simulink model "controller_full"  (R2020b)
settings: Solver=VariableStepAuto  StartTime=0.0  StopTime=10.0  RelTol=1e-3
undefined symbols (not defined in the file): K_d, K_p, params, r_des
settings Model: Creator=Danil  LastModifiedBy=Danil

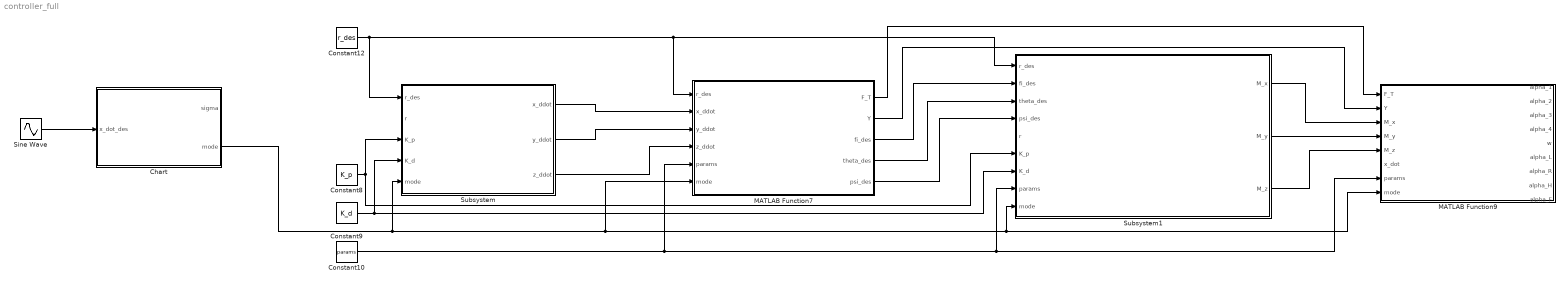
== system controller_full ==
  Chart : Stateflow chart  TreatAsAtomicUnit=on
      settings: PortSchema="{\"entries\":[{\"content\":{\"sides\":[{\"content\":{\"connectorIds\":[\"In1\"]},\"type\":\"ConnectorPlacement.EquallySpacedRectSide\",\"uuid\":\"990aaa4d-e872-427e-8bc8-a44f7de52f17\"},{\"content\":{\"connectorIds\":[\"Out2\",\"Out1\"],\"side\":\"RIGHT\"},\"type\":\"ConnectorPlacement.EquallySpacedRectSide\",\"uuid\":\"6e7ad4a8-1d47-4f26-af3c-4dfef899b5bc\"},{\"content\":{\"connectorIds\":[],\"side\":\"TOP\"},\"type\":\"ConnectorPlacement.EquallySpacedRectSide\",\"uuid\":\"20d3b10c-4783-40ca-8243-63709ccaf162\"},{\"content\":{\"connectorIds\":[],\"side\":\"HIDDEN\"},\"type\":\"ConnectorPlacement.EquallySpacedRectSide\",\"uuid\":\"c78cf433-ac9b-47b8-aa1e-24a5718d794b\"}]},\"type\":\"ConnectorPlacement.EquallySpacedConnector\",\"uuid\":\"eb598262-5703-4057-871f-faa738de211a\"}],\"packageUris\":[\"http://schema.mathworks.com/mf0/Connector/R2020b\"],\"version\":\"1.0\"}"
  Constant10 : Constant  Value=params  OutDataTypeStr=Bus: params_bus
  Constant12 : Constant  Value=r_des  OutDataTypeStr=Bus: r_des_bus
  Constant8 : Constant  Value=K_p  OutDataTypeStr=Bus: K_p_bus
  Constant9 : Constant  Value=K_d  OutDataTypeStr=Bus: K_d_bus
  MATLAB Function7 : MATLAB Function  TreatAsAtomicUnit=on
  MATLAB Function9 : MATLAB Function  TreatAsAtomicUnit=on
  Sine Wave : Sin  Amplitude=40  SampleTime=0
  Subsystem : Subsystem
  Subsystem1 : Subsystem
  wires:
  Sine Wave/1 -> Chart/1(x_dot_des)
  Subsystem1/1(M_x) -> MATLAB Function9/3(M_x)
  Subsystem1/2(M_y) -> MATLAB Function9/4(M_y)
  Subsystem1/3(M_z) -> MATLAB Function9/5(M_z)
  Constant10/1 -> MATLAB Function7/5(params), Subsystem1/8(params), MATLAB Function9/7(params)
  Constant12/1 -> Subsystem/1(r_des), MATLAB Function7/1(r_des), Subsystem1/1(r_des)
  Constant8/1 -> Subsystem/3(K_p), Subsystem1/6(K_p)
  Constant9/1 -> Subsystem/4(K_d), Subsystem1/7(K_d)
  Chart/1(mode) -> Subsystem/5(mode), MATLAB Function9/8(mode), Subsystem1/9(mode), MATLAB Function7/6(mode)
  Subsystem/1(x_ddot) -> MATLAB Function7/2(x_ddot)
  Subsystem/2(y_ddot) -> MATLAB Function7/3(y_ddot)
  Subsystem/3(z_ddot) -> MATLAB Function7/4(z_ddot)
  MATLAB Function7/5(psi_des) -> Subsystem1/4(psi_des)
  MATLAB Function7/4(theta_des) -> Subsystem1/3(theta_des)
  MATLAB Function7/3(fi_des) -> Subsystem1/2(fi_des)
  MATLAB Function7/2(Y) -> MATLAB Function9/2(Y)
  MATLAB Function7/1(F_T) -> MATLAB Function9/1(F_T)

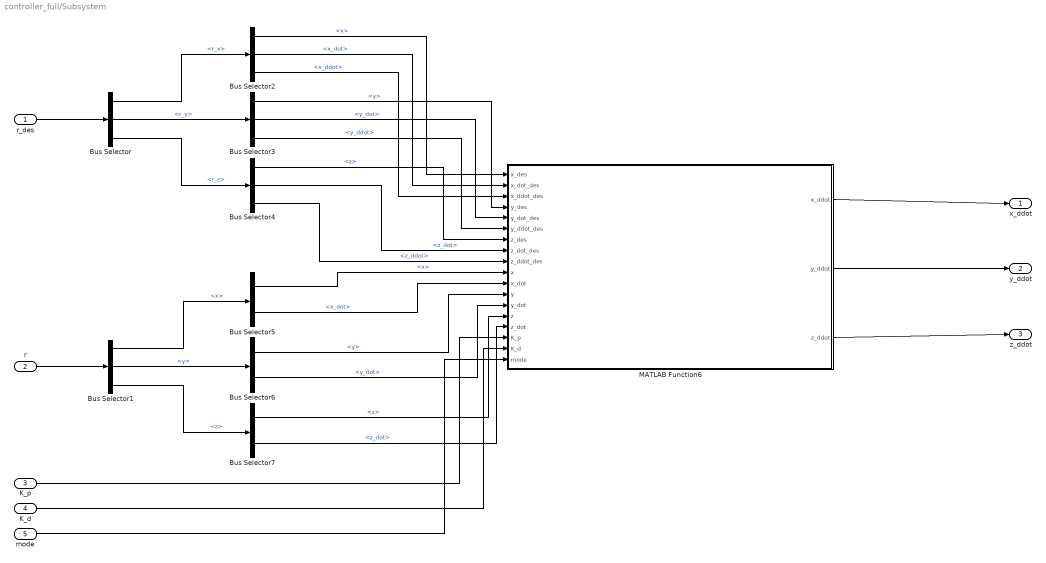
== system controller_full/Subsystem ==
  r_des : Inport
  r : Inport  Port=2
  K_p : Inport  Port=3
  K_d : Inport  Port=4
  mode : Inport  Port=5
  Bus Selector : BusSelector  OutputSignals=r_x,r_y,r_z
  Bus Selector1 : BusSelector  OutputSignals=x,y,z
  Bus Selector2 : BusSelector  OutputSignals=x,x_dot,x_ddot
  Bus Selector3 : BusSelector  OutputSignals=y,y_dot,y_ddot
  Bus Selector4 : BusSelector  OutputSignals=z,z_dot,z_ddot
  Bus Selector5 : BusSelector  OutputSignals=x,x_dot
  Bus Selector6 : BusSelector  OutputSignals=y,y_dot
  Bus Selector7 : BusSelector  OutputSignals=z,z_dot
  MATLAB Function6 : MATLAB Function  TreatAsAtomicUnit=on
  x_ddot : Outport
  y_ddot : Outport  Port=2
  z_ddot : Outport  Port=3
  wires:
  Bus Selector3/1 -> MATLAB Function6/4(y_des)  "<y>"
  Bus Selector4/3 -> MATLAB Function6/9(z_ddot_des)  "<z_ddot>"
  Bus Selector4/1 -> MATLAB Function6/7(z_des)  "<z>"
  Bus Selector/1 -> Bus Selector2/1  "<r_x>"
  Bus Selector5/2 -> MATLAB Function6/11(x_dot)  "<x_dot>"
  Bus Selector3/2 -> MATLAB Function6/5(y_dot_des)  "<y_dot>"
  Bus Selector/3 -> Bus Selector4/1  "<r_z>"
  r/1 -> Bus Selector1/1
  r_des/1 -> Bus Selector/1
  Bus Selector2/1 -> MATLAB Function6/1(x_des)  "<x>"
  Bus Selector5/1 -> MATLAB Function6/10(x)  "<x>"
  MATLAB Function6/2(y_ddot) -> y_ddot/1
  MATLAB Function6/3(z_ddot) -> z_ddot/1
  K_d/1 -> MATLAB Function6/17(K_d)
  K_p/1 -> MATLAB Function6/16(K_p)
  Bus Selector1/3 -> Bus Selector7/1  "<z>"
  Bus Selector2/2 -> MATLAB Function6/2(x_dot_des)  "<x_dot>"
  Bus Selector7/2 -> MATLAB Function6/15(z_dot)  "<z_dot>"
  MATLAB Function6/1(x_ddot) -> x_ddot/1
  Bus Selector6/1 -> MATLAB Function6/12(y)  "<y>"
  Bus Selector7/1 -> MATLAB Function6/14(z)  "<z>"
  Bus Selector4/2 -> MATLAB Function6/8(z_dot_des)  "<z_dot>"
  Bus Selector2/3 -> MATLAB Function6/3(x_ddot_des)  "<x_ddot>"
  Bus Selector1/1 -> Bus Selector5/1  "<x>"
  Bus Selector1/2 -> Bus Selector6/1  "<y>"
  Bus Selector6/2 -> MATLAB Function6/13(y_dot)  "<y_dot>"
  Bus Selector3/3 -> MATLAB Function6/6(y_ddot_des)  "<y_ddot>"
  Bus Selector/2 -> Bus Selector3/1  "<r_y>"
  mode/1 -> MATLAB Function6/18(mode)

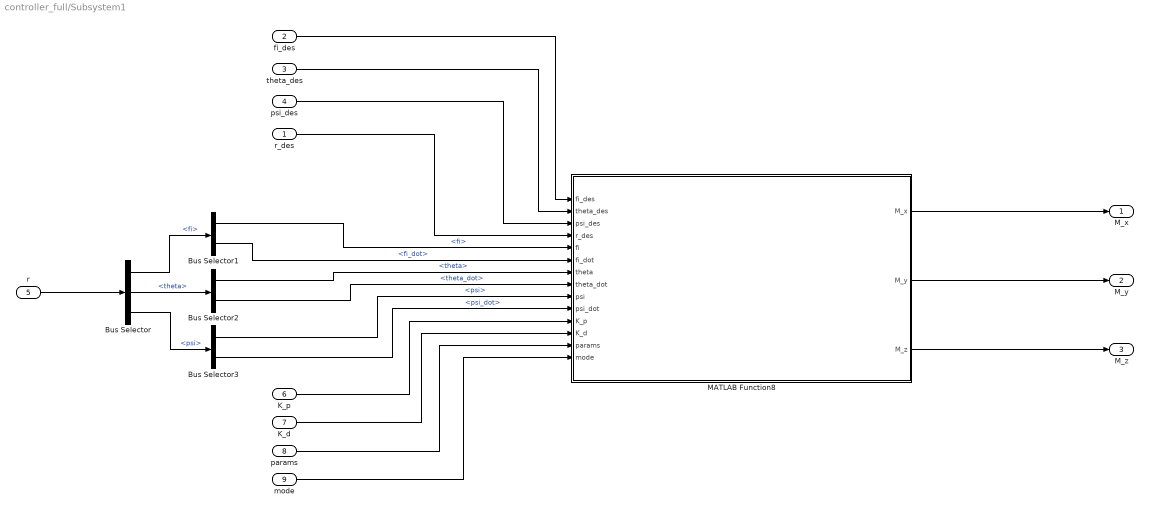
== system controller_full/Subsystem1 ==
  r_des : Inport
  fi_des : Inport  Port=2
  theta_des : Inport  Port=3
  psi_des : Inport  Port=4
  r : Inport  Port=5
  K_p : Inport  Port=6
  K_d : Inport  Port=7
  params : Inport  Port=8
  mode : Inport  Port=9
  Bus Selector : BusSelector  OutputSignals=fi,theta,psi
  Bus Selector1 : BusSelector  OutputSignals=fi,fi_dot
  Bus Selector2 : BusSelector  OutputSignals=theta,theta_dot
  Bus Selector3 : BusSelector  OutputSignals=psi,psi_dot
  MATLAB Function8 : MATLAB Function  TreatAsAtomicUnit=on
  M_x : Outport
  M_y : Outport  Port=2
  M_z : Outport  Port=3
  wires:
  Bus Selector3/1 -> MATLAB Function8/9(psi)  "<psi>"
  Bus Selector1/2 -> MATLAB Function8/6(fi_dot)  "<fi_dot>"
  Bus Selector/1 -> Bus Selector1/1  "<fi>"
  Bus Selector1/1 -> MATLAB Function8/5(fi)  "<fi>"
  r/1 -> Bus Selector/1
  MATLAB Function8/3(M_z) -> M_z/1
  MATLAB Function8/1(M_x) -> M_x/1
  MATLAB Function8/2(M_y) -> M_y/1
  Bus Selector2/2 -> MATLAB Function8/8(theta_dot)  "<theta_dot>"
  K_p/1 -> MATLAB Function8/11(K_p)
  Bus Selector2/1 -> MATLAB Function8/7(theta)  "<theta>"
  Bus Selector/2 -> Bus Selector2/1  "<theta>"
  r_des/1 -> MATLAB Function8/4(r_des)
  params/1 -> MATLAB Function8/13(params)
  psi_des/1 -> MATLAB Function8/3(psi_des)
  fi_des/1 -> MATLAB Function8/1(fi_des)
  K_d/1 -> MATLAB Function8/12(K_d)
  theta_des/1 -> MATLAB Function8/2(theta_des)
  Bus Selector3/2 -> MATLAB Function8/10(psi_dot)  "<psi_dot>"
  Bus Selector/3 -> Bus Selector3/1  "<psi>"
  mode/1 -> MATLAB Function8/14(mode)

== matlab function controller_full/MATLAB Function9 ==
  data: alpha_1 output; alpha_2 output; alpha_3 output; alpha_4 output; F_T input; Y input; w output; M_x input; M_y input; M_z input; x_dot input; params input; alpha_L output; alpha_R output; alpha_H output; alpha_F output; mode input
function [alpha_1, alpha_2, alpha_3, alpha_4, w, alpha_L, alpha_R, alpha_H, alpha_F] = fcn(F_T, Y, M_x, M_y, M_z, x_dot, params, mode)

if mode == 0
    
    alpha_1 = (1 / (4 * params.k_Y)) * (F_T + M_x + M_y + M_z) - 7;
    alpha_2 = (1 / (4 * params.k_Y)) * (F_T + M_x - M_y - M_z);
    alpha_3 = (1 / (4 * params.k_Y)) * (F_T - M_x + M_y - M_z) - 7;
    alpha_4 = (1 / (4 * params.k_Y)) * (F_T - M_x - M_y + M_z);
    
    w = params.w_0;
    alpha_L = -7;
    alpha_R = -7;
    alpha_H = 0;
    alpha_F = 0;
    
elseif mode == 1
    
    alpha_1 = 7.5;
    alpha_2 = 7.5;
    alpha_3 = 7.5;
    alpha_4 = 7.5;

    w = (50000 * F_T + 245100) / 77;

    alpha_L = (500 * M_x + 500 * Y + 102201 * params.S_k * params.rho - 14630 * params.S_k * params.rho * x_dot) / (30 * params.S_k * params.rho * (70 * x_dot - 489));
    alpha_R = - (500 * M_x - 500 * Y - 102201 * params.S_k * params.rho + 14630 * params.S_k * params.rho * x_dot) / (30 * params.S_k * params.rho * (70 * x_dot - 489));
    alpha_H = (125 * M_y) / (3 * params.S_h * params.rho * (70 * x_dot - 489));
    alpha_F = (125 * M_z) / (3 * params.S_f * params.rho * (70 * x_dot - 489));
    
end

== stateflow chart controller_full/Chart ==
  state Vertical_flight
    mode = 0
    sigma = 0
  state Horizontal_flight
    mode = 1
    sigma = 90
  (default) -> Vertical_flight
  Horizontal_flight -> Vertical_flight : [x_dot_des < 14.1]
  Vertical_flight -> Horizontal_flight : [x_dot_des > 14.1]
  data: mode output; x_dot_des input; sigma output

== matlab function controller_full/Subsystem/MATLAB Function6 ==
  data: x_des input; x_ddot output; x_dot_des input; x_ddot_des input; y_des input; y_dot_des input; y_ddot_des input; z_des input; z_dot_des input; z_ddot_des input; x input; x_dot input; y input; y_dot input; z input; z_dot input; K_p input; K_d input; y_ddot output; z_ddot output; mode input
function [x_ddot,y_ddot,z_ddot] = fcn(x_des, x_dot_des, x_ddot_des, y_des, y_dot_des, y_ddot_des, z_des, z_dot_des, z_ddot_des, ...
                                      x, x_dot, y, y_dot, z, z_dot, K_p, K_d, mode)

if mode == 0
    
    x_ddot = x_ddot_des + abs(K_d.ver.x) * (x_dot_des - x_dot) + abs(K_p.ver.x) * (x_des - x);
    y_ddot = y_ddot_des + abs(K_d.ver.y) * (y_dot_des - y_dot) + abs(K_p.ver.y) * (y_des - y);
    z_ddot = z_ddot_des + abs(K_d.ver.z) * (z_dot_des - z_dot) + abs(K_p.ver.z) * (z_des - z);

elseif mode == 1
    
    x_ddot = x_ddot_des + abs(K_d.hor.x) * (x_dot_des - x_dot) + abs(K_p.hor.x) * (x_des - x);
    y_ddot = y_ddot_des + abs(K_d.hor.y) * (y_dot_des - y_dot) + abs(K_p.hor.y) * (y_des - y);
    z_ddot = z_ddot_des + abs(K_d.hor.z) * (z_dot_des - z_dot) + abs(K_p.hor.z) * (z_des - z);
    
end

== matlab function controller_full/MATLAB Function7 ==
  data: r_des input; F_T output; Y output; fi_des output; x_ddot input; y_ddot input; z_ddot input; params input; mode input; theta_des output; psi_des output
function [F_T, Y, fi_des, theta_des, psi_des] = fcn(r_des, x_ddot, y_ddot, z_ddot, params, mode)

if mode == 0
    
    F_T = params.m * (z_ddot + params.g);
    Y = 0;

    fi_des = (1 / params.g) * (x_ddot * sin(r_des.ver.psi) - y_ddot * cos(r_des.ver.psi));
    theta_des = (1 / params.g) * (x_ddot * cos(r_des.ver.psi) + y_ddot * sin(r_des.ver.psi));
    psi_des = r_des.ver.psi;
    
elseif mode == 1
    
    %F_T = params.m * x_ddot + params.k_x * x_dot;

    F_T = params.m * x_ddot + r_des.x_dot;
    Y = params.m * params.g;

    fi_des = r_des.hor.fi;
    theta_des = (params.m / (params.k_x * r_des.x_dot)) * (y_ddot * sin(r_des.hor.fi) - z_ddot * cos(r_des.hor.fi));
    psi_des = (params.m / (params.k_x * r_des.x_dot)) * (y_ddot * cos(r_des.hor.fi) + z_ddot * sin(r_des.hor.fi));

    %theta_des = (params.m / F_T) * (y_ddot * sin(r_des.fi) - z_ddot * cos(r_des.fi));
    %psi_des = (params.m / F_T) * (y_ddot * cos(r_des.fi) + z_ddot * sin(r_des.fi));
    
end

== matlab function controller_full/Subsystem1/MATLAB Function8 ==
  data: fi_des input; theta_des input; psi_des input; r_des input; fi input; fi_dot input; theta input; theta_dot input; psi input; psi_dot input; M_x output; K_p input; K_d input; params input; M_y output; M_z output; mode input
function [M_x, M_y, M_z] = fcn(fi_des, theta_des, psi_des, r_des, fi, fi_dot, theta, theta_dot, psi, psi_dot, K_p, K_d, params, mode)

if mode == 0

    M_x = (params.ver.J_xx / params.ver.L_x) * (r_des.fi_ddot + abs(K_d.ver.fi) * (r_des.fi_dot - fi_dot) + abs(K_p.ver.fi) * (fi_des - fi));
    M_y = (params.ver.J_yy / params.ver.L_y) * (r_des.theta_ddot + abs(K_d.ver.theta) * (r_des.theta_dot - theta_dot) + abs(K_p.ver.theta) * (theta_des - theta));
    M_z = (params.ver.J_zz / params.ver.L_z) * (r_des.psi_ddot + abs(K_d.ver.psi) * (r_des.psi_dot - psi_dot) + abs(K_p.ver.psi) * (psi_des - psi));
    
elseif mode == 1
    
    M_x = (params.hor.J_xx / params.hor.L_x) * (r_des.fi_ddot + abs(K_d.hor.fi) * (r_des.fi_dot - fi_dot) + abs(K_p.hor.fi) * (fi_des - fi));
    M_y = (params.hor.J_yy / params.hor.L_y) * (r_des.theta_ddot + abs(K_d.hor.theta) * (r_des.theta_dot - theta_dot) + abs(K_p.hor.theta) * (theta_des - theta));
    M_z = (params.hor.J_zz / params.hor.L_z) * (r_des.psi_ddot + abs(K_d.hor.psi) * (r_des.psi_dot - psi_dot) + abs(K_p.hor.psi) * (psi_des - psi));
    
end
